simulink model "final_version"  (R2024b)
settings: Solver=FixedStepAuto  StartTime=0.0  StopTime=inf  RelTol=1e-3  EnableMultiTasking=on
libraries: simulink x46, stm32f4xxblockslib x20, dspstat3 x2, stm32blockslib x1
(part 1 of 2)
settings Model: STM32="{\"DigitalPortRead\":[{\"ID\":\"exam:8\"},{\"ID\":\"exam:9\"},{\"ID\":\"exam:10\"},{\"ID\":\"exam:11\"},{\"ID\":\"exam:12\"},{\"ID\":\"exam:108\"},{\"ID\":\"Bozza_V12:8\"},{\"ID\":\"Bozza_V12:9\"},{\"ID\":\"Bozza_V12:10\"},{\"ID\":\"Bozza_V12:11\"},{\"ID\":\"Bozza_V12:12\"},{\"ID\":\"Bozza_V12:108\"},{\"ID\":\"Bozza_V13:8\"},{\"ID\":\"Bozza_V13:9\"},{\"ID\":\"Bozza_V13:10\"},{\"ID\":\"Bozza_V13:11\"},{\"ID\":\"Bozza_V13:12\"},{\"ID\":\"Bozza_V13:108\"},{\"ID\":\"Bozza_V14:8\"},{\"ID\":\"Bozza_V14:9\"},{\"ID\":\"Bozza_V14:10\"},{\"ID\":\"Bozza_V14:11\"},{\"ID\":\"Bozza_V14:12\"},{\"ID\":\"Bozza_V14:108\"},{\"ID\":\"Bozza_V15:8\"},{\"ID\":\"Bozza_V15:9\"},{\"ID\":\"Bozza_V15:10\"},{\"ID\":\"Bozza_V15:11\"},{\"ID\":\"Bozza_V15:12\"},{\"ID\":\"Bozza_V15:108\"},{\"ID\":\"Bozza_V16:8\"},{\"ID\":\"Bozza_V16:9\"},{\"ID\":\"Bozza_V16:10\"},{\"ID\":\"Bozza_V16:11\"},{\"ID\":\"Bozza_V16:12\"},{\"ID\":\"Bozza_V16:108\"},{\"ID\":\"final_version:8\"},{\"ID\":\"final_version:9\"},{\"ID\":\"final_version:10\"},{\"ID\":\"final_version:11\"},{\"ID\":\"final_version:12\"},{\"ID\":\"final_version:108\"}],\"PWMOutput\":[{\"ID\":\"exam:27\"},{\"ID\":\"exam:133\"},{\"ID\":\"Bozza_V12:27\"},{\"ID\":\"Bozza_V12:133\"},{\"ID\":\"Bozza_V13:27\"},{\"ID\":\"Bozza_V13:133\"},{\"ID\":\"Bozza_V14:27\"},{\"ID\":\"Bozza_V14:133\"},{\"ID\":\"Bozza_V15:133\"},{\"ID\":\"Bozza_V15:27\"},{\"ID\":\"Bozza_V16:133\"},{\"ID\":\"Bozza_V16:27\"},{\"ID\":\"final_version:27\"},{\"ID\":\"final_version:133\"}],\"TimerCapture\":[{\"ID\":\"exam:32\"},{\"ID\":\"Bozza_V12:32\"},{\"ID\":\"Bozza_V13:32\"},{\"ID\":\"Bozza_V14:32\"},{\"ID\":\"Bozza_V15:32\"},{\"ID\":\"Bozza_V16:32\"},{\"ID\":\"final_version:32\"}],\"DigitalPortWrite\":[{\"ID\":\"exam:109\"},{\"ID\":\"exam:110\"},{\"ID\":\"exam:111\"},{\"ID\":\"exam:112\"},{\"ID\":\"exam:113\"},{\"ID\":\"exam:114\"},{\"ID\":\"exam:115\"},{\"ID\":\"exam:116\"},{\"ID\":\"exam:334\"},{\"ID\":\"exam:335\"},{\"ID\":\"exam:336\"},{\"ID\":\"exam:337\"},{\"ID\":\"exam:338\"},{\"ID\":\"exam:339\"},{\"ID\":\"exam:347\"},{\"ID\":\"exam:348\"},{\"ID\":\"exam:349\"},{\"ID\":\"exam:350\"},{\"ID\":\"exam:351\"},{\"ID\":\"exam:352\"},{\"ID\":\"exam:362\"},{\"ID\":\"exam:363\"},{\"ID\":\"exam:364\"},{\"ID\":\"exam:365\"},{\"ID\":\"exam:366\"},{\"ID\":\"exam:367\"},{\"ID\":\"exam:376\"},{\"ID\":\"exam:377\"},{\"ID\":\"exam:378\"},{\"ID\":\"exam:379\"},{\"ID\":\"exam:380\"},{\"ID\":\"exam:381\"},{\"ID\":\"exam:389\"},{\"ID\":\"exam:390\"},{\"ID\":\"exam:391\"},{\"ID\":\"exam:392\"},{\"ID\":\"exam:393\"},{\"ID\":\"exam:394\"},{\"ID\":\"exam:404\"},{\"ID\":\"exam:405\"},{\"ID\":\"exam:406\"},{\"ID\":\"exam:407\"},{\"ID\":\"exam:408\"},{\"ID\":\"exam:409\"},{\"ID\":\"exam:474\"},{\"ID\":\"exam:475\"},{\"ID\":\"exam:478\"},{\"ID\":\"Bozza_V12:475\"},{\"ID\":\"Bozza_V12:531\"},{\"ID\":\"Bozza_V12:532\"},{\"ID\":\"Bozza_V12:110\"},{\"ID\":\"Bozza_V12:111\"},{\"ID\":\"Bozza_V12:112\"},{\"ID\":\"Bozza_V12:113\"},{\"ID\":\"Bozza_V12:114\"},{\"ID\":\"Bozza_V12:115\"},{\"ID\":\"Bozza_V12:116\"},{\"ID\":\"Bozza_V12:478\"},{\"ID\":\"Bozza_V12:474\"},{\"ID\":\"Bozza_V13:110\"},{\"ID\":\"Bozza_V13:111\"},{\"ID\":\"Bozza_V13:112\"},{\"ID\":\"Bozza_V13:113\"},{\"ID\":\"Bozza_V13:114\"},{\"ID\":\"Bozza_V13:115\"},{\"ID\":\"Bozza_V13:116\"},{\"ID\":\"Bozza_V13:478\"},{\"ID\":\"Bozza_V13:475\"},{\"ID\":\"Bozza_V13:531\"},{\"ID\":\"Bozza_V13:532\"},{\"ID\":\"Bozza_V13:376\"},{\"ID\":\"Bozza_V13:377\"},{\"ID\":\"Bozza_V13:378\"},{\"ID\":\"Bozza_V13:379\"},{\"ID\":\"Bozza_V13:380\"},{\"ID\":\"Bozza_V13:381\"},{\"ID\":\"Bozza_V13:389\"},{\"ID\":\"Bozza_V13:390\"},{\"ID\":\"Bozza_V13:391\"},{\"ID\":\"Bozza_V13:392\"},{\"ID\":\"Bozza_V13:393\"},{\"ID\":\"Bozza_V13:394\"},{\"ID\":\"Bozza_V13:404\"},{\"ID\":\"Bozza_V13:405\"},{\"ID\":\"Bozza_V13:406\"},{\"ID\":\"Bozza_V13:407\"},{\"ID\":\"Bozza_V13:408\"},{\"ID\":\"Bozza_V13:409\"},{\"ID\":\"Bozza_V13:474\"},{\"ID\":\"Bozza_V13:339\"},{\"ID\":\"Bozza_V13:338\"},{\"ID\":\"Bozza_V13:337\"},{\"ID\":\"Bozza_V13:336\"},{\"ID\":\"Bozza_V13:335\"},{\"ID\":\"Bozza_V13:334\"},{\"ID\":\"Bozza_V13:352\"},{\"ID\":\"Bozza_V13:351\"},{\"ID\":\"Bozza_V13:350\"},{\"ID\":\"Bozza_V13:349\"},{\"ID\":\"Bozza_V13:348\"},{\"ID\":\"Bozza_V13:347\"},{\"ID\":\"Bozza_V13:367\"},{\"ID\":\"Bozza_V13:366\"},{\"ID\":\"Bozza_V13:365\"},{\"ID\":\"Bozza_V13:364\"},{\"ID\":\"Bozza_V13:363\"},{\"ID\":\"Bozza_V13:362\"},{\"ID\":\"Bozza_V14:110\"},{\"ID\":\"Bozza_V14:111\"},{\"ID\":\"Bozza_V14:112\"},{\"ID\":\"Bozza_V14:113\"},{\"ID\":\"Bozza_V14:114\"},{\"ID\":\"Bozza_V14:115\"},{\"ID\":\"Bozza_V14:116\"},{\"ID\":\"Bozza_V14:478\"},{\"ID\":\"Bozza_V14:474\"},{\"ID\":\"Bozza_V14:475\"},{\"ID\":\"Bozza_V14:531\"},{\"ID\":\"Bozza_V14:532\"},{\"ID\":\"Bozza_V14:334\"},{\"ID\":\"Bozza_V14:335\"},{\"ID\":\"Bozza_V14:336\"},{\"ID\":\"Bozza_V14:337\"},{\"ID\":\"Bozza_V14:338\"},{\"ID\":\"Bozza_V14:339\"},{\"ID\":\"Bozza_V14:347\"},{\"ID\":\"Bozza_V14:348\"},{\"ID\":\"Bozza_V14:349\"},{\"ID\":\"Bozza_V14:350\"},{\"ID\":\"Bozza_V14:351\"},{\"ID\":\"Bozza_V14:352\"},{\"ID\":\"Bozza_V14:362\"},{\"ID\":\"Bozza_V14:363\"},{\"ID\":\"Bozza_V14:364\"},{\"ID\":\"Bozza_V14:365\"},{\"ID\":\"Bozza_V14:366\"},{\"ID\":\"Bozza_V14:367\"},{\"ID\":\"Bozza_V14:376\"},{\"ID\":\"Bozza_V14:377\"},{\"ID\":\"Bozza_V14:378\"},{\"ID\":\"Bozza_V14:379\"},{\"ID\":\"Bozza_V14:380\"},{\"ID\":\"Bozza_V14:381\"},{\"ID\":\"Bozza_V14:389\"},{\"ID\":\"Bozza_V14:390\"},{\"ID\":\"Bozza_V14:391\"},{\"ID\":\"Bozza_V14:392\"},{\"ID\":\"Bozza_V14:393\"},{\"ID\":\"Bozza_V14:394\"},{\"ID\":\"Bozza_V14:404\"},{\"ID\":\"Bozza_V14:405\"},{\"ID\":\"Bozza_V14:406\"},{\"ID\":\"Bozza_V14:407\"},{\"ID\":\"Bozza_V14:408\"},{\"ID\":\"Bozza_V14:409\"},{\"ID\":\"Bozza_V15:110\"},{\"ID\":\"Bozza_V15:111\"},{\"ID\":\"Bozza_V15:112\"},{\"ID\":\"Bozza_V15:113\"},{\"ID\":\"Bozza_V15:114\"},{\"ID\":\"Bozza_V15:115\"},{\"ID\":\"Bozza_V15:116\"},{\"ID\":\"Bozza_V15:478\"},{\"ID\":\"Bozza_V15:474\"},{\"ID\":\"Bozza_V15:475\"},{\"ID\":\"Bozza_V15:531\"},{\"ID\":\"Bozza_V15:532\"},{\"ID\":\"Bozza_V15:376\"},{\"ID\":\"Bozza_V15:377\"},{\"ID\":\"Bozza_V15:378\"},{\"ID\":\"Bozza_V15:379\"},{\"ID\":\"Bozza_V15:380\"},{\"ID\":\"Bozza_V15:381\"},{\"ID\":\"Bozza_V15:389\"},{\"ID\":\"Bozza_V15:390\"},{\"ID\":\"Bozza_V15:391\"},{\"ID\":\"Bozza_V15:392\"},{\"ID\":\"Bozza_V15:393\"},{\"ID\":\"Bozza_V15:394\"},{\"ID\":\"Bozza_V15:404\"},{\"ID\":\"Bozza_V15:405\"},{\"ID\":\"Bozza_V15:406\"},{\"ID\":\"Bozza_V15:407\"},{\"ID\":\"Bozza_V15:408\"},{\"ID\":\"Bozza_V15:409\"},{\"ID\":\"Bozza_V16:110\"},{\"ID\":\"Bozza_V16:111\"},{\"ID\":\"Bozza_V16:112\"},{\"ID\":\"Bozza_V16:113\"},{\"ID\":\"Bozza_V16:114\"},{\"ID\":\"Bozza_V16:115\"},{\"ID\":\"Bozza_V16:116\"},{\"ID\":\"Bozza_V16:478\"},{\"ID\":\"Bozza_V16:474\"},{\"ID\":\"Bozza_V16:475\"},{\"ID\":\"Bozza_V16:531\"},{\"ID\":\"Bozza_V16:532\"},{\"ID\":\"final_version:110\"},{\"ID\":\"final_version:111\"},{\"ID\":\"final_version:112\"},{\"ID\":\"final_version:113\"},{\"ID\":\"final_version:114\"},{\"ID\":\"final_version:115\"},{\"ID\":\"final_version:116\"},{\"ID\":\"final_version:478\"},{\"ID\":\"final_version:474\"},{\"ID\":\"final_version:475\"},{\"ID\":\"final_version:531\"},{\"ID\":\"final_version:532\"}]}"  Creator=Utente  LastModifiedBy=Utente
settings SolverCC: AutoInsertRateTranBlk=on
settings OptimizationCC: DefaultParameterBehavior=Inlined  EnhancedBackFolding=on  PassReuseOutputArgsAs=Individual arguments  ZeroExternalMemoryAtStartup=off  ZeroInternalMemoryAtStartup=off  MaxStackSize=512  OptimizeBlockOrder=speed  DifferentSizesBufferReuse=on  OptimizationCustomize=off  EfficientTunableParamExpr=on
settings DebuggingCC: MultiTaskCondExecSysMsg=none  ParameterTunabilityLossMsg=error
settings HardwareCC: ProdBitPerPointer=32  ProdBitPerSizeT=32  ProdBitPerPtrDiffT=32  ProdLargestAtomicInteger=Long  ProdLargestAtomicFloat=Double  ProdWordSize=32  ProdLongLongMode=on  ProdHWDeviceType=ARM Compatible->ARM Cortex-M
settings RTWCC: Description=Embedded Coder  SystemTargetFile=ert.tlc  HardwareBoard=STM32F4xx Based  TemplateMakefile=ert_default_tmf  Toolchain=GNU Tools for ARM Embedded Processors
settings CodeAppCC: ForceParamTrailComments=on  IgnoreCustomStorageClasses=off  OperatorAnnotations=on  SimulinkDataObjDesc=on  SFDataObjDesc=on  InsertBlockDesc=on
settings ERTTargetCC: TargetLangStandard=C99 (ISO)  CodeReplacementLibrary=ARM Cortex-M  SupportContinuousTime=on  SupportVariableSizeSignals=on  ExtModeTransport=3  ExtModeStaticAlloc=on  ExtModeStaticAllocSize=2048  ExtModeMexFile=ext_xcp  ExtModeIntrfLevel=Level2 - Open

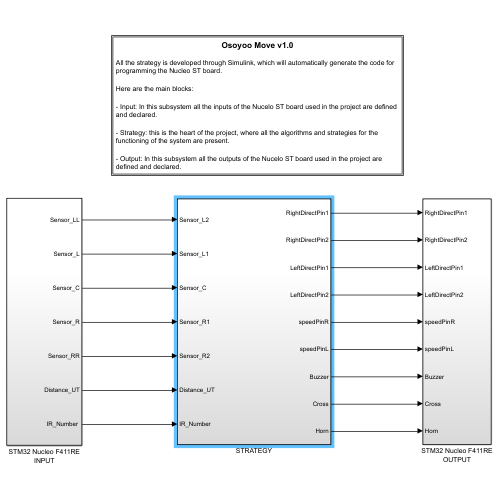
[thumbnail: Simulink's stored preview of the top-level diagram]
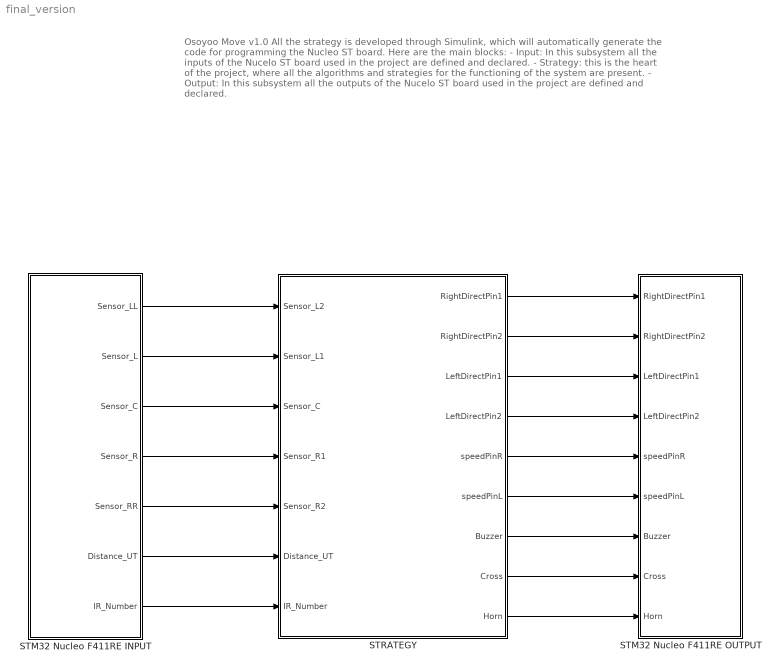
== system final_version ==
  note: Osoyoo Move v1.0
      |
      | All the strategy is developed through Simulink, which will automatically generate the code for programming the Nucleo ST board.
      |
      | Here are the main blocks:
      |
      | - Input: In this subsystem all the inputs of the Nucelo ST board used in the project are defined and declared.
      |
      | - Strategy: this is the heart of the project, where all the algorithms and strategies for the functioning of the system are present.
      |
      | - Output: In this subsystem all the outputs of the Nucelo ST board used in the project are defined and declared.
  STM32 Nucleo F411RE INPUT : Subsystem
  STM32 Nucleo F411RE OUTPUT : Subsystem
  STRATEGY : Subsystem
  wires:
  STM32 Nucleo F411RE INPUT/2(Sensor_L) -> STRATEGY/2(Sensor_L1)
  STRATEGY/8(Cross) -> STM32 Nucleo F411RE OUTPUT/8(Cross)
  STRATEGY/4(LeftDirectPin2) -> STM32 Nucleo F411RE OUTPUT/4(LeftDirectPin2)
  STM32 Nucleo F411RE INPUT/1(Sensor_LL) -> STRATEGY/1(Sensor_L2)
  STRATEGY/7(Buzzer) -> STM32 Nucleo F411RE OUTPUT/7(Buzzer)
  STRATEGY/5(speedPinR) -> STM32 Nucleo F411RE OUTPUT/5(speedPinR)
  STM32 Nucleo F411RE INPUT/6(Distance_UT) -> STRATEGY/6(Distance_UT)
  STRATEGY/6(speedPinL) -> STM32 Nucleo F411RE OUTPUT/6(speedPinL)
  STRATEGY/3(LeftDirectPin1) -> STM32 Nucleo F411RE OUTPUT/3(LeftDirectPin1)
  STM32 Nucleo F411RE INPUT/4(Sensor_R) -> STRATEGY/4(Sensor_R1)
  STM32 Nucleo F411RE INPUT/3(Sensor_C) -> STRATEGY/3(Sensor_C)
  STRATEGY/9(Horn) -> STM32 Nucleo F411RE OUTPUT/9(Horn)
  STM32 Nucleo F411RE INPUT/5(Sensor_RR) -> STRATEGY/5(Sensor_R2)
  STRATEGY/2(RightDirectPin2) -> STM32 Nucleo F411RE OUTPUT/2(RightDirectPin2)
  STRATEGY/1(RightDirectPin1) -> STM32 Nucleo F411RE OUTPUT/1(RightDirectPin1)
  STM32 Nucleo F411RE INPUT/7("IR_Number ") -> STRATEGY/7(IR_Number)

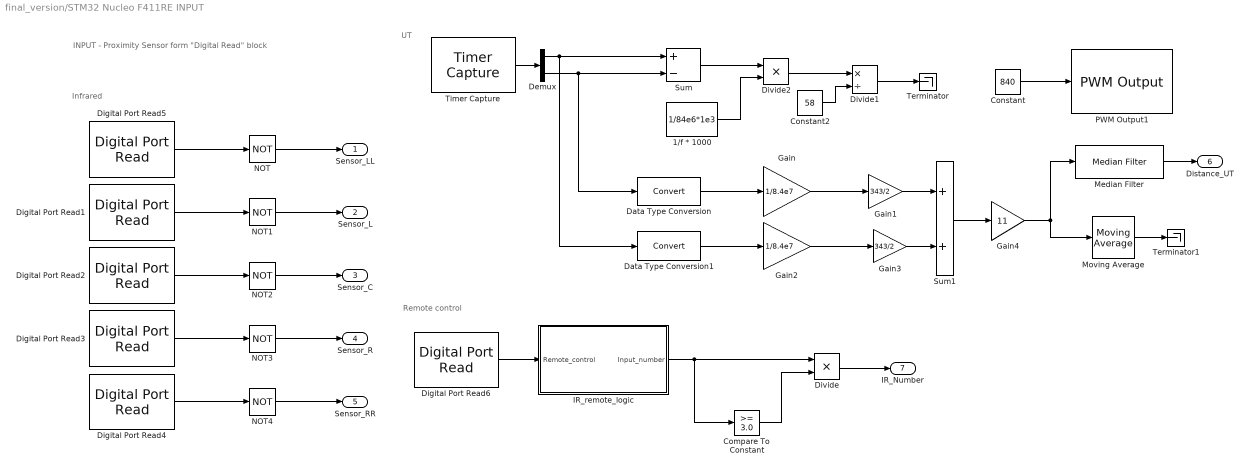
== system final_version/STM32 Nucleo F411RE INPUT ==
  note: Infrared
  note: INPUT
      |
      | - Proximity Sensor form "Digital Read" block
  note: UT
  note: Remote control
  1/f * 1000 : Constant  Value=1/84e6*1e3
  Compare To Constant : simulink/Logic and Bit Operations/Compare To Constant  relop=>=  const=3.0  OutDataTypeStr=boolean
  Constant : Constant  Value=840
  Constant2 : Constant  Value=58
  Data Type Conversion : DataTypeConversion  SaturateOnIntegerOverflow=off  RndMeth=Floor
  Data Type Conversion1 : DataTypeConversion  SaturateOnIntegerOverflow=off  RndMeth=Floor
  Demux : Demux  Outputs=2
  Digital Port Read1 : stm32f4xxblockslib/Digital Port Read  PortName=GPIOA  PinNumber=[1]  ReadOperation=on  IOAsArray=on  SampleTime=-1  EnableSimPort=off  hoistedMaskSrc=ECSoC/ECSimCodegen/Digital Port Read
  Digital Port Read2 : stm32f4xxblockslib/Digital Port Read  PortName=GPIOA  PinNumber=[4]  ReadOperation=on  IOAsArray=on  SampleTime=-1  EnableSimPort=off  hoistedMaskSrc=ECSoC/ECSimCodegen/Digital Port Read
  Digital Port Read3 : stm32f4xxblockslib/Digital Port Read  PortName=GPIOB  PinNumber=[0]  ReadOperation=on  IOAsArray=on  SampleTime=-1  EnableSimPort=off  hoistedMaskSrc=ECSoC/ECSimCodegen/Digital Port Read
  Digital Port Read4 : stm32f4xxblockslib/Digital Port Read  PortName=GPIOC  PinNumber=[1]  ReadOperation=on  IOAsArray=on  SampleTime=-1  EnableSimPort=off  hoistedMaskSrc=ECSoC/ECSimCodegen/Digital Port Read
  Digital Port Read5 : stm32f4xxblockslib/Digital Port Read  PortName=GPIOA  PinNumber=[0]  ReadOperation=on  IOAsArray=on  SampleTime=-1  EnableSimPort=off  hoistedMaskSrc=ECSoC/ECSimCodegen/Digital Port Read
  Digital Port Read6 : stm32f4xxblockslib/Digital Port Read  PortName=GPIOA  PinNumber=[6]  ReadOperation=on  IOAsArray=on  SampleTime=-1  EnableSimPort=off  hoistedMaskSrc=ECSoC/ECSimCodegen/Digital Port Read
  Divide : Product  Inputs=**
  Divide1 : Product  Inputs=*/
  Divide2 : Product  Inputs=**
  Gain : Gain  Gain=1/8.4e7
  Gain1 : Gain  Gain=343/2
  Gain2 : Gain  Gain=1/8.4e7
  Gain3 : Gain  Gain=343/2
  Gain4 : Gain  Gain=11
  IR_remote_logic : Subsystem  TreatAsAtomicUnit=on
  Median Filter : dspstat3/Median Filter  WindowLength=250  SimulateUsing=Interpreted execution
      settings: LibrarySourceBlock=|
      | dspfdesign/Median
      | Filter
  Moving Average : dspstat3/Moving Average  Method=Sliding window  ForgettingFactorPort=off  SpecifyWindowLength=on  WindowLength=40  OverlapLength=39  AllowArbitraryInputLength=off  ForgettingFactor=0.9  SimulateUsing=Interpreted execution
  NOT{,1..4} (5 alike) : Logic  Operator=NOT  IconShape=distinctive  AllPortsSameDT=off  OutDataTypeStr=boolean
  PWM Output1 : stm32f4xxblockslib/PWM Output  TimerModule=TIM2  DutycycleUnits=Counts  EnableChannel1=off  EnableChannel2=on  EnableChannel3=off  EnableChannel4=off  EnableCounterInput=off  EnableMainOutputInput=off  EnableFrequencyInput=off  SetRCAfterCE=off  OutputDirection=off  OutputMainOutputEnableStatus=off  SampleTime=0.1  EnableSimPort=off  EnableUpdateEvent=off  EnableCaptureCompare1Event=off  EnableCaptureCompare2Event=off  EnableCaptureCompare3Event=off  EnableCaptureCompare4Event=off  EnableTriggerEvent=off  EnableBreakEvent=off  ProcessorFamily=STM32F4  hoistedMaskSrc=ECSoC/ECSimCodegen/PWM Output
  Sum : Sum  Inputs=+-
  Sum1 : Sum
  Terminator : Terminator
  Terminator1 : Terminator
  Timer Capture : stm32blockslib/Timer Capture  TimerModule=TIM2  SelectedChannel=CH1  CaptureLength=2  OutputDataLength=off  OutputOverrunStatus=off  OutputDirection=off  SampleTime=-1
      settings: LibrarySourceBlock=stm32f4xxblockslib/Timer Capture
  Sensor_LL : Outport
  Sensor_L : Outport  Port=2
  Sensor_C : Outport  Port=3
  Sensor_R : Outport  Port=4
  Sensor_RR : Outport  Port=5
  Distance_UT : Outport  Port=6
  "IR_Number " : Outport  Port=7
  wires:
  NOT/1 -> Sensor_LL/1
  NOT1/1 -> Sensor_L/1
  NOT2/1 -> Sensor_C/1
  NOT3/1 -> Sensor_R/1
  NOT4/1 -> Sensor_RR/1
  Digital Port Read4/1 -> NOT4/1
  Digital Port Read3/1 -> NOT3/1
  Digital Port Read2/1 -> NOT2/1
  Digital Port Read1/1 -> NOT1/1
  Digital Port Read5/1 -> NOT/1
  Sum1/1 -> Gain4/1
  Gain4/1 -> Median Filter/1, Moving Average/1
  1/f * 1000/1 -> Divide2/2
  Sum/1 -> Divide2/1
  Gain3/1 -> Sum1/2
  Divide2/1 -> Divide1/1
  Gain1/1 -> Sum1/1
  Demux/1 -> Sum/1, Data Type Conversion1/1
  Gain/1 -> Gain1/1
  Divide1/1 -> Terminator/1
  Data Type Conversion1/1 -> Gain2/1
  Data Type Conversion/1 -> Gain/1
  Demux/2 -> Sum/2, Data Type Conversion/1
  Gain2/1 -> Gain3/1
  Timer Capture/1 -> Demux/1
  Constant2/1 -> Divide1/2
  Constant/1 -> PWM Output1/1
  Moving Average/1 -> Terminator1/1
  Digital Port Read6/1 -> IR_remote_logic/1(Remote_control)
  Divide/1 -> "IR_Number "/1
  IR_remote_logic/1(Input_number) -> Compare To Constant/1, Divide/1
  Compare To Constant/1 -> Divide/2
  Median Filter/1 -> Distance_UT/1

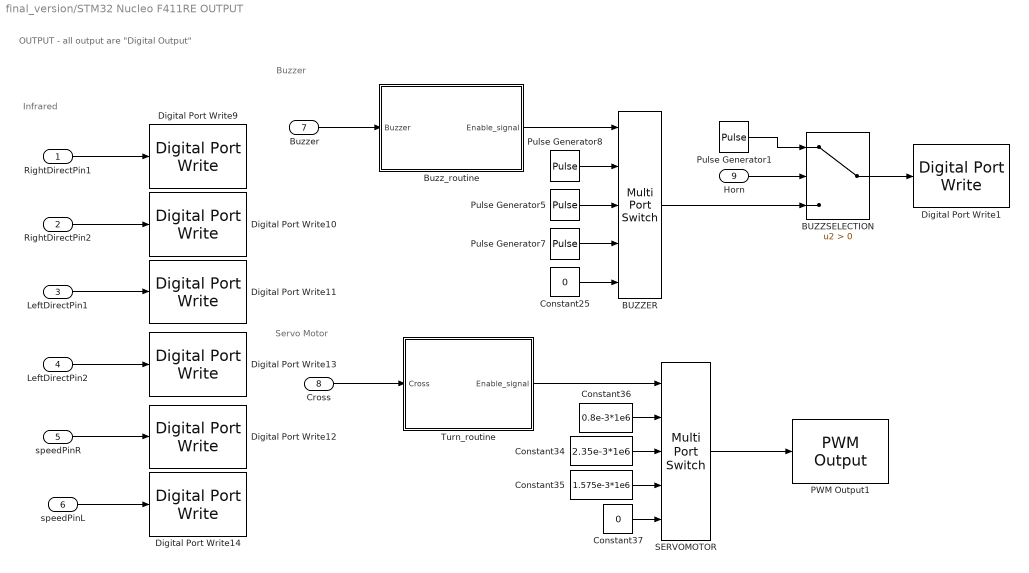
== system final_version/STM32 Nucleo F411RE OUTPUT ==
  note: Infrared
  note: OUTPUT
      |
      | - all output are "Digital Output"
  note: Buzzer
  note: Servo Motor
  RightDirectPin1 : Inport
  RightDirectPin2 : Inport  Port=2
  LeftDirectPin1 : Inport  Port=3
  LeftDirectPin2 : Inport  Port=4
  speedPinR : Inport  Port=5
  speedPinL : Inport  Port=6
  Buzzer : Inport  Port=7
  Cross : Inport  Port=8
  Horn : Inport  Port=9
  BUZZER : MultiPortSwitch  Inputs=4  SaturateOnIntegerOverflow=off  InputSameDT=off
  BUZZSELECTION : Switch  Criteria=u2 > Threshold  SaturateOnIntegerOverflow=off  InputSameDT=off
  Buzz_routine : Subsystem
  Constant25 : Constant  Value=0
  Constant34 : Constant  Value=2.35e-3*1e6
  Constant35 : Constant  Value=1.575e-3*1e6
  Constant36 : Constant  Value=0.8e-3*1e6
  Constant37 : Constant  Value=0
  Digital Port Write1 : stm32f4xxblockslib/Digital Port Write  PortName=GPIOA  PinNumber=[7]  ReadOperation=off  IOAsArray=on  EnableSimPort=off  hoistedMaskSrc=ECSoC/ECSimCodegen/Digital Port Write
  Digital Port Write10 : stm32f4xxblockslib/Digital Port Write  PortName=GPIOA  PinNumber=[9]  ReadOperation=off  IOAsArray=on  EnableSimPort=off  hoistedMaskSrc=ECSoC/ECSimCodegen/Digital Port Write
  Digital Port Write11 : stm32f4xxblockslib/Digital Port Write  PortName=GPIOC  PinNumber=[7]  ReadOperation=off  IOAsArray=on  EnableSimPort=off  hoistedMaskSrc=ECSoC/ECSimCodegen/Digital Port Write
  Digital Port Write12 : stm32f4xxblockslib/Digital Port Write  PortName=GPIOB  PinNumber=[4]  ReadOperation=off  IOAsArray=on  EnableSimPort=off  hoistedMaskSrc=ECSoC/ECSimCodegen/Digital Port Write
  Digital Port Write13 : stm32f4xxblockslib/Digital Port Write  PortName=GPIOB  PinNumber=[6]  ReadOperation=off  IOAsArray=on  EnableSimPort=off  hoistedMaskSrc=ECSoC/ECSimCodegen/Digital Port Write
  Digital Port Write14 : stm32f4xxblockslib/Digital Port Write  PortName=GPIOB  PinNumber=[10]  ReadOperation=off  IOAsArray=on  EnableSimPort=off  hoistedMaskSrc=ECSoC/ECSimCodegen/Digital Port Write
  Digital Port Write9 : stm32f4xxblockslib/Digital Port Write  PortName=GPIOA  PinNumber=[8]  ReadOperation=off  IOAsArray=on  EnableSimPort=off  hoistedMaskSrc=ECSoC/ECSimCodegen/Digital Port Write
  PWM Output1 : stm32f4xxblockslib/PWM Output  TimerModule=TIM1  DutycycleUnits=Counts  EnableChannel1=off  EnableChannel2=off  EnableChannel3=on  EnableChannel4=off  EnableCounterInput=off  EnableMainOutputInput=off  EnableFrequencyInput=off  SetRCAfterCE=off  OutputDirection=off  OutputMainOutputEnableStatus=off  SampleTime=0.1  EnableSimPort=off  EnableUpdateEvent=off  EnableCaptureCompare1Event=off  EnableCaptureCompare2Event=off  EnableCaptureCompare3Event=off  EnableCaptureCompare4Event=off  EnableTriggerEvent=off  EnableBreakEvent=off  ProcessorFamily=STM32F4  hoistedMaskSrc=ECSoC/ECSimCodegen/PWM Output
  Pulse Generator1 : DiscretePulseGenerator  PulseType=Time based  Period=0.001  PulseWidth=50
  Pulse Generator5 : DiscretePulseGenerator  PulseType=Time based  Period=1/250  PulseWidth=50
  Pulse Generator7 : DiscretePulseGenerator  PulseType=Time based  Period=1/500  PulseWidth=50
  Pulse Generator8 : DiscretePulseGenerator  PulseType=Time based  Period=0.006  PulseWidth=50
  SERVOMOTOR : MultiPortSwitch  DataPortForDefault=Additional data port  SaturateOnIntegerOverflow=off  InputSameDT=off
  Turn_routine : Subsystem
  wires:
  Pulse Generator7/1 -> BUZZER/4
  Pulse Generator5/1 -> BUZZER/3
  Pulse Generator8/1 -> BUZZER/2
  Buzz_routine/1(Enable_signal) -> BUZZER/1
  Constant25/1 -> BUZZER/5
  Buzzer/1 -> Buzz_routine/1(Buzzer)
  Constant35/1 -> SERVOMOTOR/4
  Constant37/1 -> SERVOMOTOR/5
  SERVOMOTOR/1 -> PWM Output1/1
  Constant34/1 -> SERVOMOTOR/3
  Constant36/1 -> SERVOMOTOR/2
  Cross/1 -> Turn_routine/1(Cross)
  Turn_routine/1(Enable_signal) -> SERVOMOTOR/1
  RightDirectPin2/1 -> Digital Port Write10/1
  RightDirectPin1/1 -> Digital Port Write9/1
  LeftDirectPin1/1 -> Digital Port Write11/1
  LeftDirectPin2/1 -> Digital Port Write13/1
  speedPinR/1 -> Digital Port Write12/1
  speedPinL/1 -> Digital Port Write14/1
  BUZZSELECTION/1 -> Digital Port Write1/1
  BUZZER/1 -> BUZZSELECTION/3
  Pulse Generator1/1 -> BUZZSELECTION/1
  Horn/1 -> BUZZSELECTION/2

== system final_version/STRATEGY ==
  note: STRATEGY
      |
      | The strategy is divided into two function blocks:
      |
      | 1 - "DecideDirection": within this block the algorithms that decide the direction to take according to the input sensors are implemented.
      |
      | 2 - "CalculatePins": this block defines how the outputs are to be controlled according to the desired direction.
  Sensor_L2 : Inport
  Sensor_L1 : Inport  Port=2
  Sensor_C : Inport  Port=3
  Sensor_R1 : Inport  Port=4
  Sensor_R2 : Inport  Port=5
  Distance_UT : Inport  Port=6
  IR_Number : Inport  Port=7
  CalculatePins : Subsystem
  Constant : Constant  Value=100
  DecideDirection : Subsystem
  Forward_LED_routine : Subsystem
  RightDirectPin1 : Outport
  RightDirectPin2 : Outport  Port=2
  LeftDirectPin1 : Outport  Port=3
  LeftDirectPin2 : Outport  Port=4
  speedPinR : Outport  Port=5
  speedPinL : Outport  Port=6
  Buzzer : Outport  Port=7
  Cross : Outport  Port=8
  Horn : Outport  Port=9
  wires:
  DecideDirection/6(TurnRight) -> Forward_LED_routine/6(TurnRight), CalculatePins/6(TurnRight)
  DecideDirection/3(TurnLeft) -> Forward_LED_routine/3(TurnLeft), CalculatePins/3(TurnLeft)
  Constant/1 -> CalculatePins/8("speed ")
  Sensor_R2/1 -> DecideDirection/5(Sensor_R2)
  Sensor_R1/1 -> DecideDirection/4(Sensor_R1)
  Sensor_C/1 -> DecideDirection/3(Sensor_C)
  Sensor_L1/1 -> DecideDirection/2(Sensor_L1)
  Sensor_L2/1 -> DecideDirection/1(Sensor_L2)
  CalculatePins/1("RightPin1 ") -> RightDirectPin1/1
  CalculatePins/2(RightPin2) -> RightDirectPin2/1
  CalculatePins/3(LeftPin1) -> LeftDirectPin1/1
  CalculatePins/4(LeftPin2) -> LeftDirectPin2/1
  CalculatePins/5("SpeedPin1 ") -> speedPinR/1
  CalculatePins/6(SpeedPin2) -> speedPinL/1
  DecideDirection/4(TurnSlightLeft) -> Forward_LED_routine/4(TurnSlightLeft), CalculatePins/4("TurnSlightLeft ")
  DecideDirection/8(Buzzer) -> Buzzer/1
  Distance_UT/1 -> DecideDirection/6(Distance_UT)
  DecideDirection/9(Horn) -> Horn/1
  DecideDirection/1(GoForward) -> CalculatePins/1(GoForward), Forward_LED_routine/1(GoForward)
  DecideDirection/5(TurnSlightRight) -> Forward_LED_routine/5(TurnSlightRight), CalculatePins/5(TurnSlightRight)
  DecideDirection/10(Cross) -> Cross/1
  IR_Number/1 -> DecideDirection/7(IR_Number)
  DecideDirection/7(Reverse) -> CalculatePins/7(Reverse)
  DecideDirection/2(Stop) -> Forward_LED_routine/2(Stop), CalculatePins/2(Stop)

== system final_version/STM32 Nucleo F411RE INPUT/IR_remote_logic ==
  Remote_control : Inport
  Constant : Constant
  Data Type Conversion : DataTypeConversion  OutDataTypeStr=uint8  SaturateOnIntegerOverflow=off  RndMeth=Floor
  Delay : Delay  DelayLength=400
  Divide : Product  Inputs=**
  Relational Operator : RelationalOperator  Operator=>  OutDataTypeStr=boolean  RndMeth=Simplest  InputSameDT=off
  Relational Operator1 : RelationalOperator  Operator===  OutDataTypeStr=boolean  RndMeth=Simplest  InputSameDT=off
  Sum : Sum
  Unit Delay : UnitDelay  SampleTime=-1  HasFrameUpgradeWarning=on
  Unit Delay1 : UnitDelay  SampleTime=-1  HasFrameUpgradeWarning=on
  delayed_signal : Delay  DelayLength=1500
  resetted_max : MATLAB Function  TreatAsAtomicUnit=on
  signal : Sum  Inputs=|+-
  signal_to_reset : Sum  Inputs=-+
  Input_number : Outport
  wires:
  Constant/1 -> signal/2
  Relational Operator/1 -> Data Type Conversion/1
  Unit Delay/1 -> Relational Operator/2
  Sum/1 -> signal/1, Unit Delay1/1
  Data Type Conversion/1 -> Sum/1
  Unit Delay1/1 -> Sum/2
  Remote_control/1 -> Relational Operator/1, Unit Delay/1
  delayed_signal/1 -> signal_to_reset/1
  signal/1 -> delayed_signal/1, signal_to_reset/2
  signal_to_reset/1 -> resetted_max/1(x)
  Divide/1 -> Input_number/1
  resetted_max/1(y) -> Delay/1, Relational Operator1/2, Divide/2
  Delay/1 -> Relational Operator1/1
  Relational Operator1/1 -> Divide/1

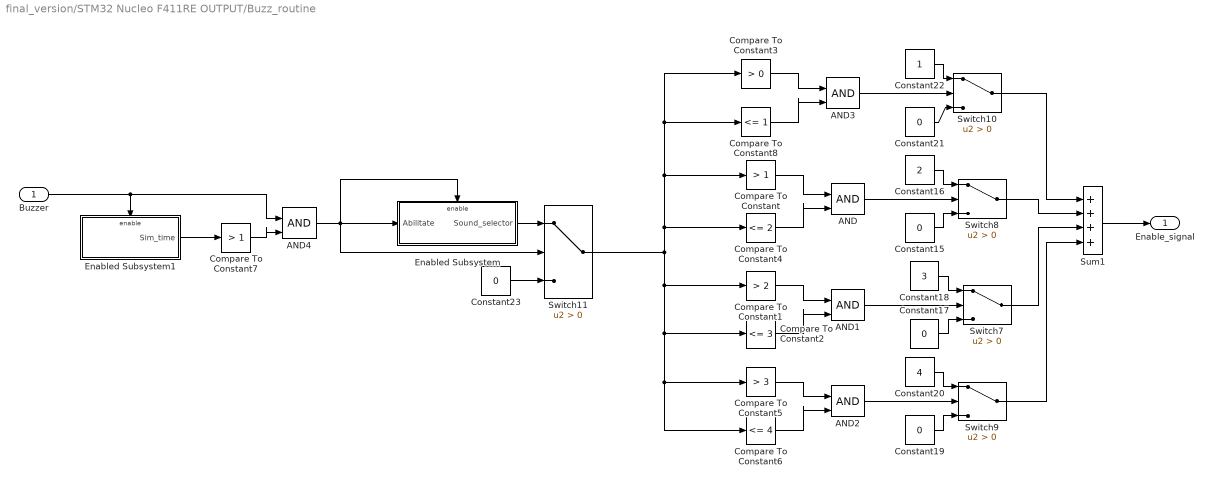
== system final_version/STM32 Nucleo F411RE OUTPUT/Buzz_routine ==
  Buzzer : Inport
  AND{,1..4} (5 alike) : Logic  IconShape=distinctive  AllPortsSameDT=off  OutDataTypeStr=boolean
  Compare To Constant : simulink/Logic and Bit Operations/Compare To Constant  relop=>  const=1  OutDataTypeStr=boolean
  Compare To Constant1 : simulink/Logic and Bit Operations/Compare To Constant  relop=>  const=2  OutDataTypeStr=boolean
  Compare To Constant2 : simulink/Logic and Bit Operations/Compare To Constant  relop=<=  const=3  OutDataTypeStr=boolean
  Compare To Constant3 : simulink/Logic and Bit Operations/Compare To Constant  relop=>  const=0  OutDataTypeStr=boolean
  Compare To Constant4 : simulink/Logic and Bit Operations/Compare To Constant  relop=<=  const=2  OutDataTypeStr=boolean
  Compare To Constant5 : simulink/Logic and Bit Operations/Compare To Constant  relop=>  const=3  OutDataTypeStr=boolean
  Compare To Constant6 : simulink/Logic and Bit Operations/Compare To Constant  relop=<=  const=4  OutDataTypeStr=boolean
  Compare To Constant7 : simulink/Logic and Bit Operations/Compare To Constant  relop=>  const=1  OutDataTypeStr=boolean
  Compare To Constant8 : simulink/Logic and Bit Operations/Compare To Constant  relop=<=  const=1  OutDataTypeStr=boolean
  Constant{15,17,19,21,23} (5 alike) : Constant  Value=0
  Constant16 : Constant  Value=2
  Constant18 : Constant  Value=3
  Constant20 : Constant  Value=4
  Constant22 : Constant
  Enabled Subsystem : Subsystem  TreatAsAtomicUnit=on
  Enabled Subsystem1 : Subsystem  TreatAsAtomicUnit=on
  Sum1 : Sum  Inputs=++++
  Switch{7..11} (5 alike) : Switch  Criteria=u2 > Threshold  SaturateOnIntegerOverflow=off  InputSameDT=off
  Enable_signal : Outport
  wires:
  AND1/1 -> Switch7/2
  Constant22/1 -> Switch10/1
  AND4/1 -> Switch11/2, Enabled Subsystem/1(Abilitate), Enabled Subsystem/Enable
  AND3/1 -> Switch10/2
  Switch10/1 -> Sum1/1
  Constant19/1 -> Switch9/3
  Constant18/1 -> Switch7/1
  AND2/1 -> Switch9/2
  Enabled Subsystem1/1(Sim_time) -> Compare To Constant7/1
  Constant15/1 -> Switch8/3
  Constant21/1 -> Switch10/3
  Compare To Constant1/1 -> AND1/1
  Buzzer/1 -> AND4/1, Enabled Subsystem1/Enable
  Switch9/1 -> Sum1/4
  Compare To Constant8/1 -> AND3/2
  Compare To Constant2/1 -> AND1/2
  Switch7/1 -> Sum1/3
  Constant23/1 -> Switch11/3
  Compare To Constant/1 -> AND/1
  Constant16/1 -> Switch8/1
  Compare To Constant7/1 -> AND4/2
  AND/1 -> Switch8/2
  Switch8/1 -> Sum1/2
  Compare To Constant6/1 -> AND2/2
  Compare To Constant4/1 -> AND/2
  Constant20/1 -> Switch9/1
  Compare To Constant3/1 -> AND3/1
  Enabled Subsystem/1(Sound_selector) -> Switch11/1
  Compare To Constant5/1 -> AND2/1
  Constant17/1 -> Switch7/3
  Sum1/1 -> Enable_signal/1
  Switch11/1 -> Compare To Constant2/1, Compare To Constant5/1, Compare To Constant6/1, Compare To Constant1/1, Compare To Constant/1, Compare To Constant8/1, Compare To Constant3/1, Compare To Constant4/1

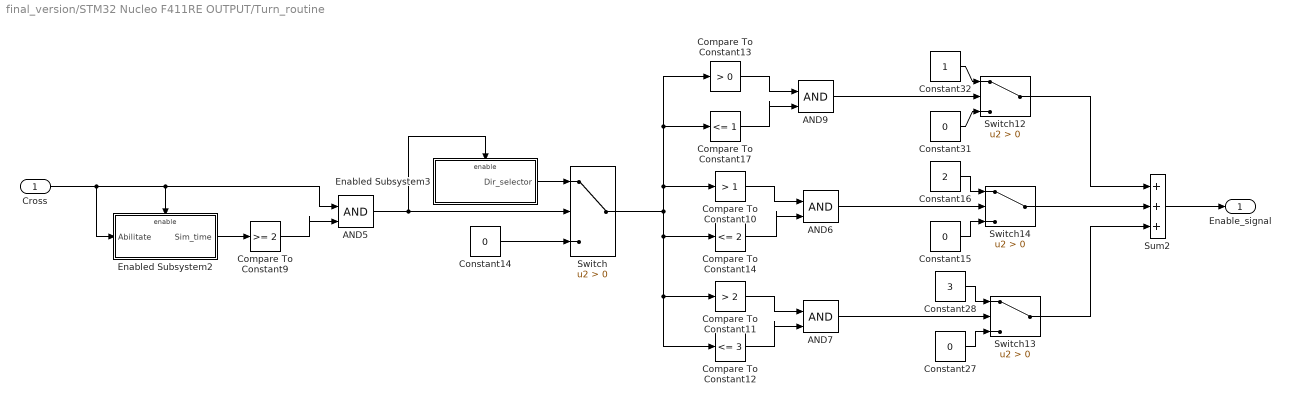
== system final_version/STM32 Nucleo F411RE OUTPUT/Turn_routine ==
  Cross : Inport
  AND{5..7,9} (4 alike) : Logic  IconShape=distinctive  AllPortsSameDT=off  OutDataTypeStr=boolean
  Compare To Constant10 : simulink/Logic and Bit Operations/Compare To Constant  relop=>  const=1  OutDataTypeStr=boolean
  Compare To Constant11 : simulink/Logic and Bit Operations/Compare To Constant  relop=>  const=2  OutDataTypeStr=boolean
  Compare To Constant12 : simulink/Logic and Bit Operations/Compare To Constant  relop=<=  const=3  OutDataTypeStr=boolean
  Compare To Constant13 : simulink/Logic and Bit Operations/Compare To Constant  relop=>  const=0  OutDataTypeStr=boolean
  Compare To Constant14 : simulink/Logic and Bit Operations/Compare To Constant  relop=<=  const=2  OutDataTypeStr=boolean
  Compare To Constant17 : simulink/Logic and Bit Operations/Compare To Constant  relop=<=  const=1  OutDataTypeStr=boolean
  Compare To Constant9 : simulink/Logic and Bit Operations/Compare To Constant  relop=>=  const=2  OutDataTypeStr=boolean
  Constant{14..15,27,31} (4 alike) : Constant  Value=0
  Constant16 : Constant  Value=2
  Constant28 : Constant  Value=3
  Constant32 : Constant
  Enabled Subsystem2 : Subsystem  TreatAsAtomicUnit=on
  Enabled Subsystem3 : Subsystem  TreatAsAtomicUnit=on
  Sum2 : Sum  Inputs=+++
  Switch{,12..14} (4 alike) : Switch  Criteria=u2 > Threshold  SaturateOnIntegerOverflow=off  InputSameDT=off
  Enable_signal : Outport
  wires:
  Constant16/1 -> Switch14/1
  Switch/1 -> Compare To Constant11/1, Compare To Constant12/1, Compare To Constant14/1, Compare To Constant10/1, Compare To Constant13/1, Compare To Constant17/1
  Constant31/1 -> Switch12/3
  Compare To Constant13/1 -> AND9/1
  Compare To Constant17/1 -> AND9/2
  Constant27/1 -> Switch13/3
  Compare To Constant12/1 -> AND7/2
  Constant14/1 -> Switch/3
  AND7/1 -> Switch13/2
  Enabled Subsystem2/1(Sim_time) -> Compare To Constant9/1
  Switch14/1 -> Sum2/2
  Switch13/1 -> Sum2/3
  Cross/1 -> Enabled Subsystem2/1(Abilitate), AND5/1, Enabled Subsystem2/Enable
  AND6/1 -> Switch14/2
  AND5/1 -> Enabled Subsystem3/Enable, Switch/2
  Compare To Constant14/1 -> AND6/2
  Constant28/1 -> Switch13/1
  Compare To Constant10/1 -> AND6/1
  Switch12/1 -> Sum2/1
  Constant32/1 -> Switch12/1
  AND9/1 -> Switch12/2
  Compare To Constant9/1 -> AND5/2
  Compare To Constant11/1 -> AND7/1
  Constant15/1 -> Switch14/3
  Enabled Subsystem3/1(Dir_selector) -> Switch/1
  Sum2/1 -> Enable_signal/1

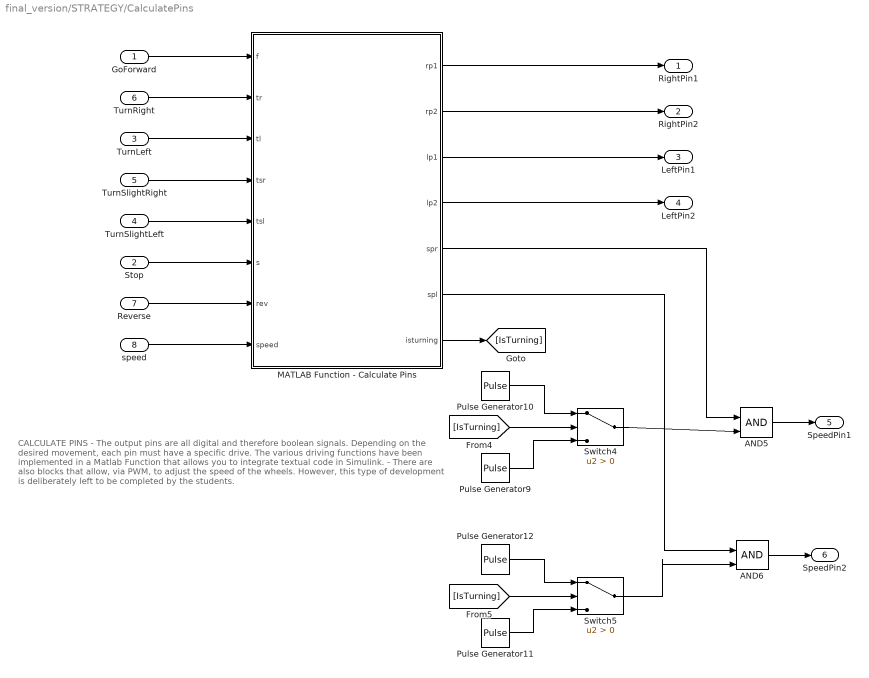
== system final_version/STRATEGY/CalculatePins ==
  note: CALCULATE PINS
      |
      | - The output pins are all digital and therefore boolean signals. Depending on the desired movement, each pin must have a specific drive. The various driving functions have been implemented in a Matlab Function that allows you to integrate textual code in Simulink.
      |
      | - There are also blocks that allow, via PWM, to adjust the speed of the wheels. However, this type of development is deliberately left to be completed by the students.
  GoForward : Inport
  Stop : Inport  Port=2
  TurnLeft : Inport  Port=3
  "TurnSlightLeft " : Inport  Port=4
  TurnSlightRight : Inport  Port=5
  TurnRight : Inport  Port=6
  Reverse : Inport  Port=7
  "speed " : Inport  Port=8
  AND5 : Logic  IconShape=distinctive  AllPortsSameDT=off  OutDataTypeStr=boolean
  AND6 : Logic  IconShape=distinctive  AllPortsSameDT=off  OutDataTypeStr=boolean
  MATLAB Function - Calculate Pins : MATLAB Function  TreatAsAtomicUnit=on
  Pulse Generator{9..12} (4 alike) : DiscretePulseGenerator  PulseType=Time based  Period=.01  PulseWidth=25  SampleTime=-1
  Switch4 : Switch  Criteria=u2 > Threshold  SaturateOnIntegerOverflow=off  InputSameDT=off
  Switch5 : Switch  Criteria=u2 > Threshold  SaturateOnIntegerOverflow=off  InputSameDT=off
  "RightPin1 " : Outport
  RightPin2 : Outport  Port=2
  LeftPin1 : Outport  Port=3
  LeftPin2 : Outport  Port=4
  "SpeedPin1 " : Outport  Port=5
  SpeedPin2 : Outport  Port=6
  wires:
  TurnRight/1 -> MATLAB Function - Calculate Pins/2(tr)
  TurnSlightRight/1 -> MATLAB Function - Calculate Pins/4(tsr)
  "TurnSlightLeft "/1 -> MATLAB Function - Calculate Pins/5(tsl)
  TurnLeft/1 -> MATLAB Function - Calculate Pins/3(tl)
  GoForward/1 -> MATLAB Function - Calculate Pins/1(f)
  Stop/1 -> MATLAB Function - Calculate Pins/6(s)
  "speed "/1 -> MATLAB Function - Calculate Pins/8(speed)
  Pulse Generator10/1 -> Switch4/1
  Pulse Generator9/1 -> Switch4/3
  Switch4/1 -> AND5/2
  [IsTurning] -> Switch4/2
  AND5/1 -> "SpeedPin1 "/1
  Pulse Generator12/1 -> Switch5/1
  Pulse Generator11/1 -> Switch5/3
  Switch5/1 -> AND6/2
  [IsTurning] -> Switch5/2
  AND6/1 -> SpeedPin2/1
  MATLAB Function - Calculate Pins/7(isturning) -> [IsTurning]
  MATLAB Function - Calculate Pins/6(spl) -> AND6/1
  MATLAB Function - Calculate Pins/5(spr) -> AND5/1
  MATLAB Function - Calculate Pins/4(lp2) -> LeftPin2/1
  MATLAB Function - Calculate Pins/3(lp1) -> LeftPin1/1
  MATLAB Function - Calculate Pins/2(rp2) -> RightPin2/1
  MATLAB Function - Calculate Pins/1(rp1) -> "RightPin1 "/1
  Reverse/1 -> MATLAB Function - Calculate Pins/7(rev)

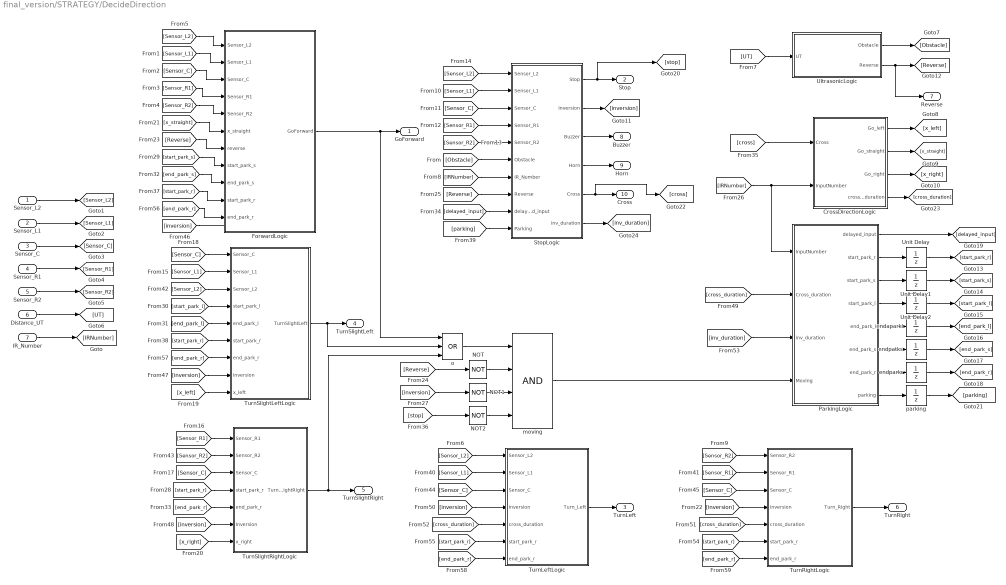
== system final_version/STRATEGY/DecideDirection ==
  Sensor_L2 : Inport
  Sensor_L1 : Inport  Port=2
  Sensor_C : Inport  Port=3
  Sensor_R1 : Inport  Port=4
  Sensor_R2 : Inport  Port=5
  Distance_UT : Inport  Port=6
  IR_Number : Inport  Port=7
  CrossDirectionLogic : Subsystem
  ForwardLogic : Subsystem
  NOT : Logic  Operator=NOT  IconShape=distinctive  AllPortsSameDT=off  OutDataTypeStr=boolean
  NOT1 : Logic  Operator=NOT  IconShape=distinctive  AllPortsSameDT=off  OutDataTypeStr=boolean
  NOT2 : Logic  Operator=NOT  IconShape=distinctive  AllPortsSameDT=off  OutDataTypeStr=boolean
  ParkingLogic : Subsystem
  StopLogic : Subsystem
  TurnLeftLogic : Subsystem
  TurnRightLogic : Subsystem
  TurnSlightLeftLogic : Subsystem
  TurnSlightRightLogic : Subsystem
  UltrasonicLogic : Subsystem
  Unit Delay : UnitDelay  SampleTime=-1  HasFrameUpgradeWarning=on
  Unit Delay1 : UnitDelay  SampleTime=-1  HasFrameUpgradeWarning=on
  Unit Delay2 : UnitDelay  SampleTime=-1  HasFrameUpgradeWarning=on
  endaparkl : UnitDelay  SampleTime=-1  HasFrameUpgradeWarning=on
  endparkr : UnitDelay  SampleTime=-1  HasFrameUpgradeWarning=on
  endpatks : UnitDelay  SampleTime=-1  HasFrameUpgradeWarning=on
  moving : Logic  Inputs=4  IconShape=distinctive  AllPortsSameDT=off  OutDataTypeStr=boolean
  o : Logic  Operator=OR  Inputs=3  IconShape=distinctive  AllPortsSameDT=off  OutDataTypeStr=boolean
  parking : UnitDelay  SampleTime=-1  HasFrameUpgradeWarning=on
  GoForward : Outport
  Stop : Outport  Port=2
  TurnLeft : Outport  Port=3
  TurnSlightLeft : Outport  Port=4
  TurnSlightRight : Outport  Port=5
  TurnRight : Outport  Port=6
  Reverse : Outport  Port=7
  Buzzer : Outport  Port=8
  Horn : Outport  Port=9
  Cross : Outport  Port=10
  wires:
  TurnSlightLeftLogic/1(TurnSlightLeft) -> o/2, TurnSlightLeft/1
  TurnSlightRightLogic/1(TurnSlightRight) -> o/3, TurnSlightRight/1
  StopLogic/5(Cross) -> [cross], Cross/1
  ForwardLogic/1(GoForward) -> o/1, GoForward/1
  [IRNumber] -> CrossDirectionLogic/2(InputNumber), ParkingLogic/1(InputNumber)
  ParkingLogic/2(start_park_r) -> Unit Delay/1
  ParkingLogic/3(start_park_s) -> Unit Delay1/1
  ParkingLogic/4("start_park_l ") -> Unit Delay2/1
  Unit Delay/1 -> [start_park_r]
  Unit Delay1/1 -> [start_park_s]
  Unit Delay2/1 -> [start_park_l]
  o/1 -> moving/1
  [Reverse] -> NOT/1
  NOT/1 -> moving/2
  NOT1/1 -> moving/3
  [inversion] -> NOT1/1
  moving/1 -> ParkingLogic/4(Moving)
  CrossDirectionLogic/1(Go_left) -> [x_left]
  CrossDirectionLogic/2(Go_straight) -> [x_straight]
  CrossDirectionLogic/3(Go_right) -> [x_right]
  Sensor_L2/1 -> [Sensor_L2]
  Sensor_L1/1 -> [Sensor_L1]
  Sensor_C/1 -> [Sensor_C]
  Sensor_R1/1 -> [Sensor_R1]
  Sensor_R2/1 -> [Sensor_R2]
  Distance_UT/1 -> [UT]
  IR_Number/1 -> [IRNumber]
  [Sensor_R1] -> TurnSlightRightLogic/1(Sensor_R1)
  [Sensor_C] -> TurnSlightRightLogic/3(Sensor_C)
  [start_park_r] -> TurnSlightRightLogic/4(start_park_r)
  [Sensor_C] -> TurnSlightLeftLogic/1(Sensor_C)
  [Sensor_L1] -> TurnSlightLeftLogic/2(Sensor_L1)
  [start_park_l] -> TurnSlightLeftLogic/4(start_park_l)
  [Sensor_L2] -> StopLogic/1(Sensor_L2)
  [Sensor_L1] -> StopLogic/2(Sensor_L1)
  [Sensor_C] -> StopLogic/3(Sensor_C)
  [Sensor_R1] -> StopLogic/4(Sensor_R1)
  [Sensor_R2] -> StopLogic/5(Sensor_R2)
  [Obstacle] -> StopLogic/6(Obstacle)
  [IRNumber] -> StopLogic/7(IR_Number)
  [Reverse] -> StopLogic/8(Reverse)
  StopLogic/2(Inversion) -> [inversion]
  StopLogic/3(Buzzer) -> Buzzer/1
  StopLogic/4(Horn) -> Horn/1
  [Sensor_L2] -> ForwardLogic/1(Sensor_L2)
  [Sensor_L1] -> ForwardLogic/2(Sensor_L1)
  [Sensor_C] -> ForwardLogic/3(Sensor_C)
  [Sensor_R1] -> ForwardLogic/4(Sensor_R1)
  [Sensor_R2] -> ForwardLogic/5(Sensor_R2)
  [x_straight] -> ForwardLogic/6(x_straight)
  [Reverse] -> ForwardLogic/7(reverse)
  [start_park_s] -> ForwardLogic/8(start_park_s)
  endparkr/1 -> [end_park_r]
  endpatks/1 -> [end_park_s]
  endaparkl/1 -> [end_park_l]
  ParkingLogic/5(end_park_l) -> endaparkl/1
  ParkingLogic/6(end_park_s) -> endpatks/1
  ParkingLogic/7(end_park_r) -> endparkr/1
  [end_park_l] -> TurnSlightLeftLogic/5(end_park_l)
  [end_park_s] -> ForwardLogic/9(end_park_s)
  [end_park_r] -> TurnSlightRightLogic/5(end_park_r)
  ParkingLogic/1(delayed_input) -> [delayed_input]
  [delayed_input] -> StopLogic/9(delayed_input)
  [stop] -> NOT2/1
  NOT2/1 -> moving/4
  [start_park_r] -> ForwardLogic/10(start_park_r)
  [start_park_r] -> TurnSlightLeftLogic/6(start_park_r)
  [parking] -> StopLogic/10(Parking)
  StopLogic/1(Stop) -> Stop/1, [stop]
  parking/1 -> [parking]
  ParkingLogic/8(parking) -> parking/1
  UltrasonicLogic/2(Reverse) -> [Reverse], Reverse/1
  [UT] -> UltrasonicLogic/1(UT)
  UltrasonicLogic/1(Obstacle) -> [Obstacle]
  [cross] -> CrossDirectionLogic/1(Cross)
  [Sensor_L2] -> TurnSlightLeftLogic/3(Sensor_L2)
  [Sensor_R2] -> TurnSlightRightLogic/2(Sensor_R2)
  [Sensor_L2] -> TurnLeftLogic/1(Sensor_L2)
  [Sensor_L1] -> TurnLeftLogic/2(Sensor_L1)
  [x_left] -> TurnSlightLeftLogic/9(x_left)
  TurnLeftLogic/1(Turn_Left) -> TurnLeft/1
  [Sensor_C] -> TurnLeftLogic/3(Sensor_C)
  [Sensor_R2] -> TurnRightLogic/1(Sensor_R2)
  [Sensor_R1] -> TurnRightLogic/2(Sensor_R1)
  [inversion] -> TurnRightLogic/4(inversion)
  [x_right] -> TurnSlightRightLogic/7(x_right)
  TurnRightLogic/1(Turn_Right) -> TurnRight/1
  [Sensor_C] -> TurnRightLogic/3(Sensor_C)
  [inversion] -> ?
  [inversion] -> TurnSlightLeftLogic/8(Inversion)
  [inversion] -> TurnSlightRightLogic/6(Inversion)
  [inversion] -> TurnLeftLogic/4(Inversion)
  CrossDirectionLogic/4(cross_duration) -> [cross_duration]
  [cross_duration] -> ParkingLogic/2(Cross_duration)
  [cross_duration] -> TurnRightLogic/5(cross_duration)
  [cross_duration] -> TurnLeftLogic/5(cross_duration)
  StopLogic/6(inv_duration) -> [inv_duration]
  [inv_duration] -> ParkingLogic/3(inv_duration)
  [start_park_r] -> TurnRightLogic/6(start_park_r)
  [start_park_r] -> TurnLeftLogic/6(start_park_r)
  [end_park_r] -> ForwardLogic/11(end_park_r)
  [end_park_r] -> TurnSlightLeftLogic/7(end_park_r)
  [end_park_r] -> TurnLeftLogic/7(end_park_r)
  [end_park_r] -> TurnRightLogic/7(end_park_r)

== system final_version/STRATEGY/Forward_LED_routine ==
  GoForward : Inport
  Stop : Inport  Port=2
  TurnLeft : Inport  Port=3
  TurnSlightLeft : Inport  Port=4
  TurnSlightRight : Inport  Port=5
  TurnRight : Inport  Port=6
  ABILITATE_LED : Logic  IconShape=distinctive  AllPortsSameDT=off  OutDataTypeStr=boolean
  Compare To Constant : simulink/Logic and Bit Operations/Compare To Constant  relop=~=  const=1  OutDataTypeStr=boolean
  Compare To Constant1 : simulink/Logic and Bit Operations/Compare To Constant  relop=~=  const=2  OutDataTypeStr=boolean
  Compare To Constant2 : simulink/Logic and Bit Operations/Compare To Constant  relop=~=  const=3.0  OutDataTypeStr=boolean
  Constant23 : Constant  Value=0
  Enabled Subsystem : Subsystem  TreatAsAtomicUnit=on
  Green_LED : stm32f4xxblockslib/Digital Port Write  PortName=GPIOC  PinNumber=[5]  ReadOperation=off  IOAsArray=on  EnableSimPort=off  hoistedMaskSrc=ECSoC/ECSimCodegen/Digital Port Write
  LED_Selector : Switch  Criteria=u2 > Threshold  SaturateOnIntegerOverflow=off  InputSameDT=off
  NOT : Logic  Operator=NOT  IconShape=distinctive  AllPortsSameDT=off  OutDataTypeStr=boolean
  OR : Logic  Operator=OR  Inputs=5  IconShape=distinctive  AllPortsSameDT=off  OutDataTypeStr=boolean
  Red_LED : stm32f4xxblockslib/Digital Port Write  PortName=GPIOC  PinNumber=[6]  ReadOperation=off  IOAsArray=on  EnableSimPort=off  hoistedMaskSrc=ECSoC/ECSimCodegen/Digital Port Write
  White_LED : stm32f4xxblockslib/Digital Port Write  PortName=GPIOC  PinNumber=[9]  ReadOperation=off  IOAsArray=on  EnableSimPort=off  hoistedMaskSrc=ECSoC/ECSimCodegen/Digital Port Write
  wires:
  Enabled Subsystem/1(LED_selector) -> LED_Selector/1
  Constant23/1 -> LED_Selector/3
  LED_Selector/1 -> Compare To Constant/1, Compare To Constant1/1, Compare To Constant2/1
  GoForward/1 -> OR/1
  TurnSlightRight/1 -> OR/4
  TurnSlightLeft/1 -> OR/3
  TurnLeft/1 -> OR/2
  TurnRight/1 -> OR/5
  Compare To Constant2/1 -> Green_LED/1
  Compare To Constant/1 -> White_LED/1
  Compare To Constant1/1 -> Red_LED/1
  OR/1 -> ABILITATE_LED/1
  ABILITATE_LED/1 -> Enabled Subsystem/Enable, LED_Selector/2
  Stop/1 -> NOT/1
  NOT/1 -> ABILITATE_LED/2

== system final_version/STM32 Nucleo F411RE OUTPUT/Buzz_routine/Enabled Subsystem ==
  Abilitate : Inport
  Enable : EnablePort  StatesWhenEnabling=reset
  Constant1 : Constant  Value=4
  Constant3 : Constant  Value=0
  Data Type Conversion1 : DataTypeConversion  OutDataTypeStr=uint16  SaturateOnIntegerOverflow=off  RndMeth=Floor
  Mod : Math  Operator=rem
  Pulse Generator1 : DiscretePulseGenerator  PulseType=Time based  Period=0.05  PulseWidth=50
  Relational Operator1 : RelationalOperator  Operator=>  OutDataTypeStr=boolean  RndMeth=Simplest  InputSameDT=off
  Sum : Sum
  Switch : Switch  Criteria=u2 > Threshold  SaturateOnIntegerOverflow=off  InputSameDT=off
  Unit Delay : UnitDelay  SampleTime=-1  HasFrameUpgradeWarning=on
  Unit Delay1 : UnitDelay  SampleTime=-1  HasFrameUpgradeWarning=on
  Sound_selector : Outport
  wires:
  Mod/1 -> Sound_selector/1
  Constant1/1 -> Mod/2
  Unit Delay/1 -> Relational Operator1/2
  Relational Operator1/1 -> Data Type Conversion1/1
  Unit Delay1/1 -> Sum/2
  Data Type Conversion1/1 -> Sum/1
  Sum/1 -> Mod/1, Unit Delay1/1
  Switch/1 -> Unit Delay/1, Relational Operator1/1
  Pulse Generator1/1 -> Switch/1
  Abilitate/1 -> Switch/2
  Constant3/1 -> Switch/3

== system final_version/STM32 Nucleo F411RE OUTPUT/Buzz_routine/Enabled Subsystem1 ==
  Buzzer : EnablePort  StatesWhenEnabling=reset
  Constant2 : Constant
  Data Type Conversion1 : DataTypeConversion  OutDataTypeStr=uint16  SaturateOnIntegerOverflow=off  RndMeth=Floor
  Pulse Generator1 : DiscretePulseGenerator  PulseType=Time based  Period=0.2  PulseWidth=50
  Relational Operator1 : RelationalOperator  Operator=>  OutDataTypeStr=boolean  RndMeth=Simplest  InputSameDT=off
  Sum : Sum
  Sum1 : Sum  Inputs=|+-
  Unit Delay : UnitDelay  SampleTime=-1  HasFrameUpgradeWarning=on
  Unit Delay1 : UnitDelay  SampleTime=-1  HasFrameUpgradeWarning=on
  Sim_time : Outport
  wires:
  Sum1/1 -> Sim_time/1
  Relational Operator1/1 -> Data Type Conversion1/1
  Data Type Conversion1/1 -> Sum/1
  Unit Delay1/1 -> Sum/2
  Constant2/1 -> Sum1/2
  Unit Delay/1 -> Relational Operator1/2
  Sum/1 -> Sum1/1, Unit Delay1/1
  Pulse Generator1/1 -> Unit Delay/1, Relational Operator1/1

== system final_version/STM32 Nucleo F411RE OUTPUT/Turn_routine/Enabled Subsystem2 ==
  Abilitate : Inport
  Enable : EnablePort  StatesWhenEnabling=reset
  Constant : Constant  Value=0
  Data Type Conversion : DataTypeConversion  OutDataTypeStr=uint16  SaturateOnIntegerOverflow=off  RndMeth=Floor
  Pulse Generator : DiscretePulseGenerator  PulseType=Time based  Period=0.1/2  PulseWidth=50
  Relational Operator : RelationalOperator  Operator=>  OutDataTypeStr=boolean  RndMeth=Simplest  InputSameDT=off
  Sum : Sum
  Switch : Switch  Criteria=u2 > Threshold  SaturateOnIntegerOverflow=off  InputSameDT=off
  Unit Delay : UnitDelay  SampleTime=-1  HasFrameUpgradeWarning=on
  Unit Delay1 : UnitDelay  SampleTime=-1  HasFrameUpgradeWarning=on
  Sim_time : Outport
  wires:
  Unit Delay1/1 -> Sum/2
  Unit Delay/1 -> Relational Operator/2
  Data Type Conversion/1 -> Sum/1
  Sum/1 -> Sim_time/1, Unit Delay1/1
  Relational Operator/1 -> Data Type Conversion/1
  Switch/1 -> Unit Delay/1, Relational Operator/1
  Pulse Generator/1 -> Switch/1
  Abilitate/1 -> Switch/2
  Constant/1 -> Switch/3

== system final_version/STM32 Nucleo F411RE OUTPUT/Turn_routine/Enabled Subsystem3 ==
  Enable : EnablePort  StatesWhenEnabling=reset
  Data Type Conversion1 : DataTypeConversion  OutDataTypeStr=uint16  SaturateOnIntegerOverflow=off  RndMeth=Floor
  Pulse Generator1 : DiscretePulseGenerator  PulseType=Time based  Period=0.1  PulseWidth=50
  Relational Operator1 : RelationalOperator  Operator=>  OutDataTypeStr=boolean  RndMeth=Simplest  InputSameDT=off
  Sum : Sum
  Unit Delay : UnitDelay  SampleTime=-1  HasFrameUpgradeWarning=on
  Unit Delay1 : UnitDelay  SampleTime=-1  HasFrameUpgradeWarning=on
  Dir_selector : Outport
  wires:
  Unit Delay1/1 -> Sum/2
  Data Type Conversion1/1 -> Sum/1
  Unit Delay/1 -> Relational Operator1/2
  Pulse Generator1/1 -> Unit Delay/1, Relational Operator1/1
  Sum/1 -> Dir_selector/1, Unit Delay1/1
  Relational Operator1/1 -> Data Type Conversion1/1

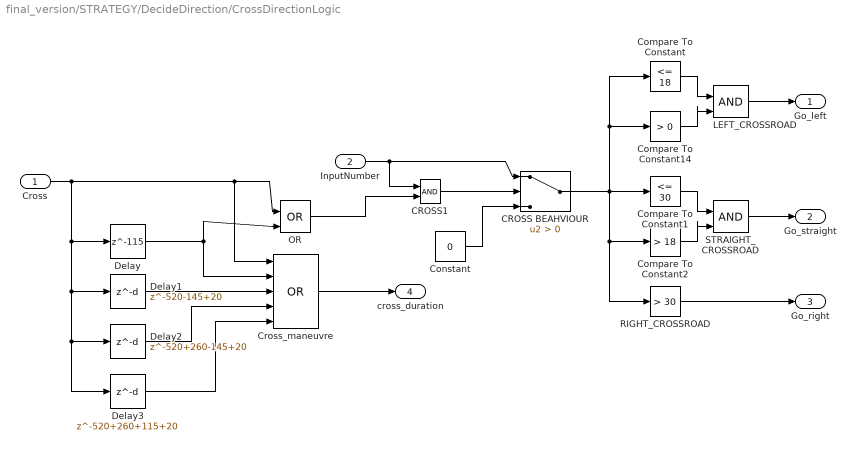
== system final_version/STRATEGY/DecideDirection/CrossDirectionLogic ==
  Cross : Inport
  InputNumber : Inport  Port=2
  "CROSS BEAHVIOUR " : Switch  Criteria=u2 > Threshold  SaturateOnIntegerOverflow=off  InputSameDT=off
  CROSS1 : Logic  IconShape=distinctive  AllPortsSameDT=off  OutDataTypeStr=boolean
  Compare To Constant : simulink/Logic and Bit Operations/Compare To Constant  relop=<=  const=18  OutDataTypeStr=boolean
  Compare To Constant1 : simulink/Logic and Bit Operations/Compare To Constant  relop=<=  const=30  OutDataTypeStr=boolean
  Compare To Constant14 : simulink/Logic and Bit Operations/Compare To Constant  relop=>  const=0  OutDataTypeStr=boolean
  Compare To Constant2 : simulink/Logic and Bit Operations/Compare To Constant  relop=>  const=18  OutDataTypeStr=boolean
  Constant : Constant  Value=0
  Cross_maneuvre : Logic  Operator=OR  Inputs=5  IconShape=distinctive  AllPortsSameDT=off  OutDataTypeStr=boolean
  Delay : Delay  DelayLength=115
  Delay1 : Delay  DelayLength=520-145+20
  Delay2 : Delay  DelayLength=520+260-145+20
  Delay3 : Delay  DelayLength=520+260+115+20
  LEFT_CROSSROAD : Logic  IconShape=distinctive  AllPortsSameDT=off  OutDataTypeStr=boolean
  OR : Logic  Operator=OR  IconShape=distinctive  AllPortsSameDT=off  OutDataTypeStr=boolean
  RIGHT_CROSSROAD : simulink/Logic and Bit Operations/Compare To Constant  relop=>  const=30  OutDataTypeStr=boolean
  STRAIGHT_CROSSROAD : Logic  IconShape=distinctive  AllPortsSameDT=off  OutDataTypeStr=boolean
  Go_left : Outport
  Go_straight : Outport  Port=2
  Go_right : Outport  Port=3
  cross_duration : Outport  Port=4
  wires:
  Compare To Constant/1 -> LEFT_CROSSROAD/1
  LEFT_CROSSROAD/1 -> Go_left/1
  Compare To Constant14/1 -> LEFT_CROSSROAD/2
  RIGHT_CROSSROAD/1 -> Go_right/1
  InputNumber/1 -> "CROSS BEAHVIOUR "/1, CROSS1/1
  CROSS1/1 -> "CROSS BEAHVIOUR "/2
  Compare To Constant2/1 -> STRAIGHT_CROSSROAD/2
  STRAIGHT_CROSSROAD/1 -> Go_straight/1
  Compare To Constant1/1 -> STRAIGHT_CROSSROAD/1
  Cross/1 -> Delay3/1, Delay2/1, Delay1/1, Delay/1, Cross_maneuvre/1, OR/1
  Constant/1 -> "CROSS BEAHVIOUR "/3
  "CROSS BEAHVIOUR "/1 -> Compare To Constant2/1, RIGHT_CROSSROAD/1, Compare To Constant1/1, Compare To Constant14/1, Compare To Constant/1
  Delay/1 -> OR/2, Cross_maneuvre/2
  Cross_maneuvre/1 -> cross_duration/1
  Delay1/1 -> Cross_maneuvre/3
  Delay2/1 -> Cross_maneuvre/4
  Delay3/1 -> Cross_maneuvre/5
  OR/1 -> CROSS1/2

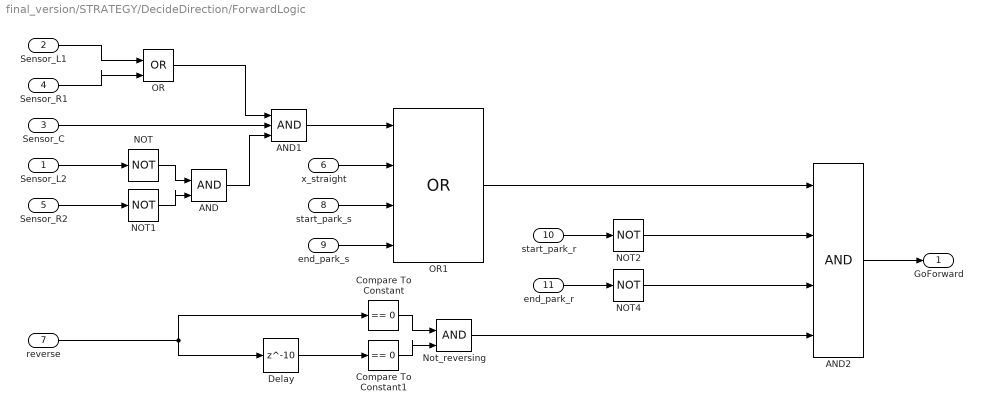
== system final_version/STRATEGY/DecideDirection/ForwardLogic ==
  Sensor_L2 : Inport
  Sensor_L1 : Inport  Port=2
  Sensor_C : Inport  Port=3
  Sensor_R1 : Inport  Port=4
  Sensor_R2 : Inport  Port=5
  x_straight : Inport  Port=6
  reverse : Inport  Port=7
  start_park_s : Inport  Port=8
  end_park_s : Inport  Port=9
  start_park_r : Inport  Port=10
  end_park_r : Inport  Port=11
  AND : Logic  IconShape=distinctive  AllPortsSameDT=off  OutDataTypeStr=boolean
  AND1 : Logic  Inputs=3  IconShape=distinctive  AllPortsSameDT=off  OutDataTypeStr=boolean
  AND2 : Logic  Inputs=4  IconShape=distinctive  AllPortsSameDT=off  OutDataTypeStr=boolean
  Compare To Constant : simulink/Logic and Bit Operations/Compare To Constant  relop===  const=0  OutDataTypeStr=boolean
  Compare To Constant1 : simulink/Logic and Bit Operations/Compare To Constant  relop===  const=0  OutDataTypeStr=boolean
  Delay : Delay  DelayLength=10
  NOT{,1..2,4} (4 alike) : Logic  Operator=NOT  IconShape=distinctive  AllPortsSameDT=off  OutDataTypeStr=boolean
  Not_reversing : Logic  IconShape=distinctive  AllPortsSameDT=off  OutDataTypeStr=boolean
  OR : Logic  Operator=OR  IconShape=distinctive  AllPortsSameDT=off  OutDataTypeStr=boolean
  OR1 : Logic  Operator=OR  Inputs=4  IconShape=distinctive  AllPortsSameDT=off  OutDataTypeStr=boolean
  GoForward : Outport
  wires:
  Sensor_L2/1 -> NOT/1
  Sensor_R2/1 -> NOT1/1
  NOT/1 -> AND/1
  NOT1/1 -> AND/2
  AND/1 -> AND1/3
  Sensor_C/1 -> AND1/2
  Sensor_R1/1 -> OR/2
  Sensor_L1/1 -> OR/1
  OR/1 -> AND1/1
  AND1/1 -> OR1/1
  x_straight/1 -> OR1/2
  AND2/1 -> GoForward/1
  OR1/1 -> AND2/1
  Delay/1 -> Compare To Constant1/1
  Compare To Constant/1 -> Not_reversing/1
  Compare To Constant1/1 -> Not_reversing/2
  reverse/1 -> Delay/1, Compare To Constant/1
  start_park_s/1 -> OR1/3
  end_park_s/1 -> OR1/4
  NOT2/1 -> AND2/2
  start_park_r/1 -> NOT2/1
  end_park_r/1 -> NOT4/1
  Not_reversing/1 -> AND2/4
  NOT4/1 -> AND2/3
